simulink model "ejercicio7_09_02_17"  (R2013a)
settings: Solver=ode45  StartTime=0.0  StopTime=10.0  RelTol=1e-3
libraries: dspsrcs4 x3, simulink x3
settings Model: Creator=Miguel  LastModifiedBy=Miguel

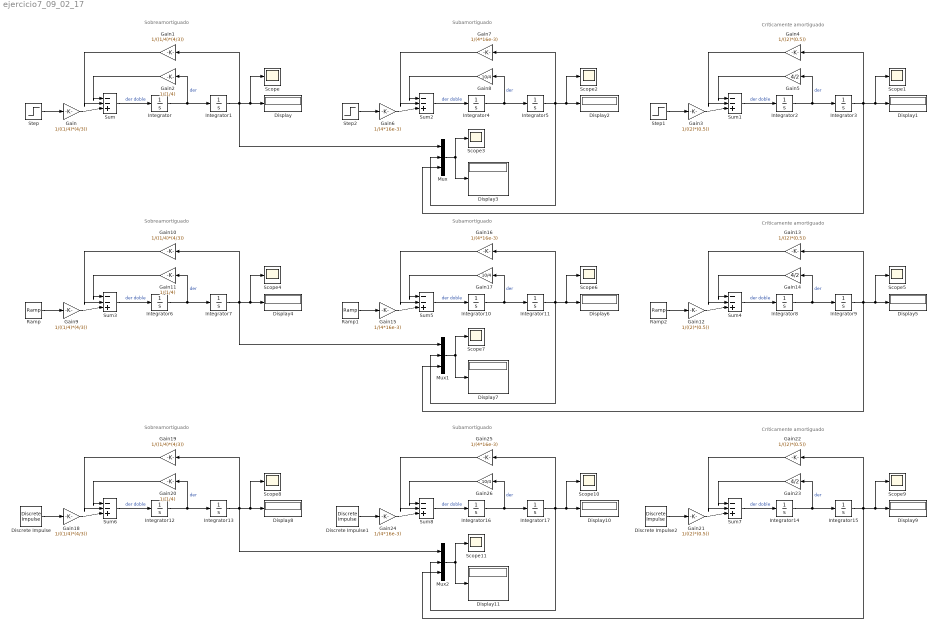
== system ejercicio7_09_02_17 ==
  note: Críticamente amortiguado
  note: Sobreamortiguado
  note: Subamortiguado
  note: Críticamente amortiguado
  note: Sobreamortiguado
  note: Subamortiguado
  note: Críticamente amortiguado
  note: Sobreamortiguado
  note: Subamortiguado
  Discrete Impulse : dspsrcs4/Discrete  Impulse  Delay=0  SampleTime=1  FrameSample=1  dataType=double  isSigned=on  wordLen=16  udDataType=sfix(16)  fracBitsMode=Best precision  numFracBits=15  OutDataTypeStr=double  LastOutDataTypeStr=double
  Discrete Impulse1 : dspsrcs4/Discrete  Impulse  Delay=0  SampleTime=1  FrameSample=1  dataType=double  isSigned=on  wordLen=16  udDataType=sfix(16)  fracBitsMode=Best precision  numFracBits=15  OutDataTypeStr=double  LastOutDataTypeStr=double
  Discrete Impulse2 : dspsrcs4/Discrete  Impulse  Delay=0  SampleTime=1  FrameSample=1  dataType=double  isSigned=on  wordLen=16  udDataType=sfix(16)  fracBitsMode=Best precision  numFracBits=15  OutDataTypeStr=double  LastOutDataTypeStr=double
  Display{,1..11} (12 alike) : Display
  Gain{,1,9..10,18..19} (6 alike) : Gain  Gain=1/((1/4)*(4/3))
  Gain11 : Gain  Gain=1/(1/4)
  Gain{3..4,12..13,21..22} (6 alike) : Gain  Gain=1/((2)*(0.5))
  Gain14 : Gain  Gain=4/2
  Gain{6..7,15..16,24..25} (6 alike) : Gain  Gain=1/(4*16e-3)
  Gain17 : Gain  Gain=10/4
  Gain2 : Gain  Gain=1/(1/4)
  Gain20 : Gain  Gain=1/(1/4)
  Gain23 : Gain  Gain=4/2
  Gain26 : Gain  Gain=10/4
  Gain5 : Gain  Gain=4/2
  Gain8 : Gain  Gain=10/4
  Integrator{,1..17} (18 alike) : Integrator
  Mux : Mux  Inputs=3
  Mux1 : Mux  Inputs=3
  Mux2 : Mux  Inputs=3
  Ramp : simulink/Sources/Ramp  slope=1  start=0  X0=0
  Ramp1 : simulink/Sources/Ramp  slope=1  start=0  X0=0
  Ramp2 : simulink/Sources/Ramp  slope=1  start=0  X0=0
  Scope{,1..11} (12 alike) : Scope
      Scope10 settings: SaveName=ScopeData8
      Scope11 settings: ShowLegends=on  SaveName=ScopeData9
      Scope2 settings: SaveName=ScopeData2
      Scope3 settings: ShowLegends=on  SaveName=ScopeData3
      Scope4 settings: SaveName=ScopeData4
      Scope5 settings: SaveName=ScopeData5
      Scope6 settings: SaveName=ScopeData6
      Scope7 settings: ShowLegends=on  SaveName=ScopeData7
      Scope8 settings: SaveName=ScopeData10
      Scope9 settings: SaveName=ScopeData11
  Step : Step  SampleTime=0
  Step1 : Step  SampleTime=0
  Step2 : Step  SampleTime=0
  Sum{,1..8} (9 alike) : Sum  Inputs=|--+
  wires:
  Integrator/1 -> Gain2/1, Integrator1/1  "der"
  Gain/1 -> Sum/3
  Sum/1 -> Integrator/1  "der doble"
  Integrator1/1 -> Mux/1, Display/1, Scope/1, Gain1/1
  Step/1 -> Gain/1
  Gain1/1 -> Sum/2
  Gain2/1 -> Sum/1
  Integrator2/1 -> Gain5/1, Integrator3/1  "der"
  Gain3/1 -> Sum1/3
  Sum1/1 -> Integrator2/1  "der doble"
  Integrator3/1 -> Mux/3, Display1/1, Scope1/1, Gain4/1
  Step1/1 -> Gain3/1
  Gain4/1 -> Sum1/2
  Gain5/1 -> Sum1/1
  Integrator4/1 -> Gain8/1, Integrator5/1  "der"
  Gain6/1 -> Sum2/3
  Sum2/1 -> Integrator4/1  "der doble"
  Integrator5/1 -> Mux/2, Display2/1, Scope2/1, Gain7/1
  Step2/1 -> Gain6/1
  Gain7/1 -> Sum2/2
  Gain8/1 -> Sum2/1
  Mux/1 -> Display3/1, Scope3/1
  Integrator6/1 -> Gain11/1, Integrator7/1  "der"
  Gain9/1 -> Sum3/3
  Sum3/1 -> Integrator6/1  "der doble"
  Integrator7/1 -> Mux1/1, Display4/1, Scope4/1, Gain10/1
  Ramp/1 -> Gain9/1
  Gain10/1 -> Sum3/2
  Gain11/1 -> Sum3/1
  Integrator8/1 -> Gain14/1, Integrator9/1  "der"
  Gain12/1 -> Sum4/3
  Sum4/1 -> Integrator8/1  "der doble"
  Integrator9/1 -> Mux1/3, Display5/1, Scope5/1, Gain13/1
  Ramp2/1 -> Gain12/1
  Gain13/1 -> Sum4/2
  Gain14/1 -> Sum4/1
  Integrator10/1 -> Gain17/1, Integrator11/1  "der"
  Gain15/1 -> Sum5/3
  Sum5/1 -> Integrator10/1  "der doble"
  Integrator11/1 -> Mux1/2, Display6/1, Scope6/1, Gain16/1
  Ramp1/1 -> Gain15/1
  Gain16/1 -> Sum5/2
  Gain17/1 -> Sum5/1
  Mux1/1 -> Display7/1, Scope7/1
  Integrator12/1 -> Gain20/1, Integrator13/1  "der"
  Gain18/1 -> Sum6/3
  Sum6/1 -> Integrator12/1  "der doble"
  Integrator13/1 -> Mux2/1, Display8/1, Scope8/1, Gain19/1
  Discrete Impulse/1 -> Gain18/1
  Gain19/1 -> Sum6/2
  Gain20/1 -> Sum6/1
  Integrator14/1 -> Gain23/1, Integrator15/1  "der"
  Gain21/1 -> Sum7/3
  Sum7/1 -> Integrator14/1  "der doble"
  Integrator15/1 -> Mux2/3, Display9/1, Scope9/1, Gain22/1
  Discrete Impulse2/1 -> Gain21/1
  Gain22/1 -> Sum7/2
  Gain23/1 -> Sum7/1
  Integrator16/1 -> Gain26/1, Integrator17/1  "der"
  Gain24/1 -> Sum8/3
  Sum8/1 -> Integrator16/1  "der doble"
  Integrator17/1 -> Mux2/2, Display10/1, Scope10/1, Gain25/1
  Discrete Impulse1/1 -> Gain24/1
  Gain25/1 -> Sum8/2
  Gain26/1 -> Sum8/1
  Mux2/1 -> Display11/1, Scope11/1
